simulink model "allmodes"  (Simulink 7.4)
settings: Solver=ode23tb  StartTime=0.0  StopTime=inf  MaxStep=1e-4  RelTol=1e-4
undefined symbols (not defined in the file): Ion, Lithium
libraries: powerlib x185, electricdrivelib x21, powerlib_extras x19, simulink x5
(part 5 of 7)

== system allmodes/vechicle units/vechicle-8 ==
  C1v8 : powerlib/Elements/Series RLC Branch  DialogController=POWERSYS.PowerSysDialog  PhysicalDomain=powersysdomain  SubClassName=unknown  LeftPortType=p1  RightPortType=p1  LConnTagsString=__new0  RConnTagsString=__new0  BranchType=C  Resistance=0.75  Inductance=1e-3  SetiL0=off  InitialCurrent=0  Capacitance=33e-6  Setx0=on  InitialVoltage=0  Measurements=Branch voltage and current
  Demux3 : Demux  Outputs=3
  Demux4 : Demux  Outputs=3
  IGBT20 : Subsystem
  IGBT21 : Subsystem
  L11v8 : powerlib/Elements/Series RLC Branch  DialogController=POWERSYS.PowerSysDialog  PhysicalDomain=powersysdomain  SubClassName=unknown  LeftPortType=p1  RightPortType=p1  LConnTagsString=__new0  RConnTagsString=__new0  BranchType=RL  Resistance=0.001  Inductance=0.0033  SetiL0=off  InitialCurrent=0  Capacitance=1e-6  Setx0=off  InitialVoltage=0  Measurements=Branch voltage and current
  L22v8 : powerlib/Elements/Series RLC Branch  DialogController=POWERSYS.PowerSysDialog  PhysicalDomain=powersysdomain  SubClassName=unknown  LeftPortType=p1  RightPortType=p1  LConnTagsString=__new0  RConnTagsString=__new0  BranchType=RL  Resistance=0.001  Inductance=1.2e-4  SetiL0=off  InitialCurrent=0  Capacitance=1e-6  Setx0=off  InitialVoltage=0  Measurements=Branch current
  Multimeter3 : powerlib/Measurements/Multimeter  SystemSampleTime=-1  PhasorSimulation=off  OutputType=Complex  sel=[41 112 113]  L=119  Gain=[1 1 1]  yselected={'Ub: vechicle units/vechicle-8/C1v8','Ib: vechicle units/vechicle-8/L11v8','Ib: vechicle units/vechicle-8/L22v8'};  PSBOutputType=1  PSBequivalent=0  AxesSetting=[0,0.1,-100,100]  Display=0  SavedBlockNames=-11
  v-8 : electricdrivelib/Extra Sources/Battery  DialogController=POWERSYS.PowerSysDialog  SystemSampleTime=-1  BatType=Lithium-Ion  ShowDetailedParameters=off  NomV=200  NomQ=30  SOC=50  PresetModel=on  MaxQ=30  FullV=232.7974  Dis_rate=13.0435  R=0.066667  Normal_OP=27.1304  expZone="[216.0772      1.473913]"  Dis_Char=off  current=[1.5 70]  Units=Ampere-hour  Batt_Tr=30
  +ve : PMIOPort  Port=1  Side=Left
  -ve : PMIOPort  Port=2  Side=Left
  tag scope: ISUIMv8=global, IbSUIMv8=global, Ibatv8=global, VbSUIMv8=global, VcSUIMv8=global, socv8=global
  wires:
  Demux3/1 -> [VcSUIMv8]
  Demux3/3 -> [IbSUIMv8]
  Demux3/2 -> [ISUIMv8]
  Multimeter3/1 -> Demux3/1
  Demux4/3 -> [VbSUIMv8]
  Demux4/2 -> [Ibatv8]
  Demux4/1 -> [socv8]
  v-8/1 -> Demux4/1
  connections:
  +ve/RConn1 -- IGBT20/RConn1
  L22v8/RConn1 -- v-8/LConn1
  IGBT21/RConn1 -- IGBT20/RConn2 -- L11v8/LConn1
  IGBT21/RConn2 -- -ve/RConn1 -- C1v8/RConn1 -- v-8/LConn2
  L11v8/RConn1 -- L22v8/LConn1 -- C1v8/LConn1

== system allmodes/vechicle units/vechicle-9 ==
  C1v9 : powerlib/Elements/Series RLC Branch  DialogController=POWERSYS.PowerSysDialog  PhysicalDomain=powersysdomain  SubClassName=unknown  LeftPortType=p1  RightPortType=p1  LConnTagsString=__new0  RConnTagsString=__new0  BranchType=C  Resistance=0.75  Inductance=1e-3  SetiL0=off  InitialCurrent=0  Capacitance=33e-6  Setx0=on  InitialVoltage=0  Measurements=Branch voltage and current
  Demux3 : Demux  Outputs=3
  Demux4 : Demux  Outputs=3
  IGBT20 : Subsystem
  IGBT21 : Subsystem
  L11v9 : powerlib/Elements/Series RLC Branch  DialogController=POWERSYS.PowerSysDialog  PhysicalDomain=powersysdomain  SubClassName=unknown  LeftPortType=p1  RightPortType=p1  LConnTagsString=__new0  RConnTagsString=__new0  BranchType=RL  Resistance=0.001  Inductance=0.0033  SetiL0=off  InitialCurrent=0  Capacitance=1e-6  Setx0=off  InitialVoltage=0  Measurements=Branch voltage and current
  L22v9 : powerlib/Elements/Series RLC Branch  DialogController=POWERSYS.PowerSysDialog  PhysicalDomain=powersysdomain  SubClassName=unknown  LeftPortType=p1  RightPortType=p1  LConnTagsString=__new0  RConnTagsString=__new0  BranchType=RL  Resistance=0.001  Inductance=1.2e-4  SetiL0=off  InitialCurrent=0  Capacitance=1e-6  Setx0=off  InitialVoltage=0  Measurements=Branch current
  Multimeter3 : powerlib/Measurements/Multimeter  SystemSampleTime=-1  PhasorSimulation=off  OutputType=Complex  sel=[43 115 116]  L=119  Gain=[1 1 1]  yselected={'Ub: vechicle units/vechicle-9/C1v9','Ib: vechicle units/vechicle-9/L11v9','Ib: vechicle units/vechicle-9/L22v9'};  PSBOutputType=1  PSBequivalent=0  AxesSetting=[0,0.1,-100,100]  Display=0  SavedBlockNames=-11
  v-9 : electricdrivelib/Extra Sources/Battery  DialogController=POWERSYS.PowerSysDialog  SystemSampleTime=-1  BatType=Lithium-Ion  ShowDetailedParameters=off  NomV=200  NomQ=30  SOC=50  PresetModel=on  MaxQ=30  FullV=232.7974  Dis_rate=13.0435  R=0.066667  Normal_OP=27.1304  expZone="[216.0772      1.473913]"  Dis_Char=off  current=[1.5 70]  Units=Ampere-hour  Batt_Tr=30
  +ve : PMIOPort  Port=1  Side=Left
  -ve : PMIOPort  Port=2  Side=Left
  tag scope: ISUIMv9=global, IbSUIMv9=global, Ibatv9=global, VbSUIMv9=global, VcSUIMv9=global, socv9=global
  wires:
  v-9/1 -> Demux4/1
  Demux4/1 -> [socv9]
  Demux4/2 -> [Ibatv9]
  Demux4/3 -> [VbSUIMv9]
  Multimeter3/1 -> Demux3/1
  Demux3/2 -> [ISUIMv9]
  Demux3/3 -> [IbSUIMv9]
  Demux3/1 -> [VcSUIMv9]
  connections:
  C1v9/LConn1 -- L22v9/LConn1 -- L11v9/RConn1
  v-9/LConn2 -- C1v9/RConn1 -- -ve/RConn1 -- IGBT21/RConn2
  L11v9/LConn1 -- IGBT20/RConn2 -- IGBT21/RConn1
  L22v9/RConn1 -- v-9/LConn1
  +ve/RConn1 -- IGBT20/RConn1

== system allmodes/CONTROLLER/AC/DC/AC controller/I-D REF ==
  Vdc_ref : Inport
  Vdc : Inport  Port=2
  Io : Inport  Port=3
  Gain1 : Gain  Gain=1/10  ParameterDataType=fixdt(1, 16)  ParameterScaling=2^0  OutDataType=fixdt(1, 16)  OutScaling=2^0
  Gain2 : Gain  Gain=1/0.7*0.25*0.5  ParameterDataType=fixdt(1, 16)  ParameterScaling=2^0  OutDataType=fixdt(1, 16)  OutScaling=2^0
  Gain3 : Gain  ParameterDataType=fixdt(1, 16)  ParameterScaling=2^0  OutDataType=fixdt(1, 16)  OutScaling=2^0
  Gain8 : Gain  Gain=10*5  ParameterDataType=fixdt(1, 16)  ParameterScaling=2^0  OutDataType=fixdt(1, 16)  OutScaling=2^0
  Integrator : Integrator
  Saturation : Saturate  UpperLimit=10000  LowerLimit=-10000  OutDataType=fixdt(1, 16)  OutScaling=2^0
  Sum : Sum  Inputs=+|+|+  OutDataType=fixdt(1, 16)  OutScaling=2^0
  Sum1 : Sum  Inputs=|+-  OutDataType=fixdt(1, 16)  OutScaling=2^0
  Sum3 : Sum  Inputs=|+-  OutDataType=fixdt(1, 16)  OutScaling=2^0
  Sum4 : Sum  Inputs=++|  OutDataType=fixdt(1, 16)  OutScaling=2^0
  Id_ref : Outport
  wires:
  Sum1/1 -> Gain8/1, Sum4/2
  Sum/1 -> Sum3/2, Saturation/1
  Vdc_ref/1 -> Sum1/1
  Vdc/1 -> Sum1/2
  Saturation/1 -> Id_ref/1, Sum3/1
  Sum3/1 -> Gain1/1
  Gain1/1 -> Sum4/1
  Integrator/1 -> Sum/2
  Gain8/1 -> Sum/3
  Gain2/1 -> Sum/1
  Gain3/1 -> Integrator/1
  Sum4/1 -> Gain3/1
  Io/1 -> Gain2/1

== system allmodes/CONTROLLER/AC/DC/AC controller/abc-dq ==
  In1 : Inport
  Demux : Demux  Outputs=3
  Discrete Virtual PLL : powerlib_extras/Discrete  Control Blocks/Discrete Virtual PLL  DialogController=POWERSYS.PowerSysDialog  SystemSampleTime=-1  Freq=60  Phase=0  Ts=50e-6
  Mux : Mux  Inputs=2
  abc_to_dq0 ransformation : powerlib_extras/Measurements/abc_to_dq0 Transformation  DialogController=POWERSYS.PowerSysDialog  SystemSampleTime=-1
  d : Outport
  wires:
  In1/1 -> abc_to_dq0 ransformation/1
  Discrete Virtual PLL/2 -> abc_to_dq0 ransformation/2
  abc_to_dq0 ransformation/1 -> Demux/1
  Demux/1 -> Mux/1
  Demux/2 -> Mux/2
  Mux/1 -> d/1

== system allmodes/CONTROLLER/AC/DC/AC controller/abc-dq2 ==
  In1 : Inport
  Demux : Demux  Outputs=3
  Discrete Virtual PLL : powerlib_extras/Discrete  Control Blocks/Discrete Virtual PLL  DialogController=POWERSYS.PowerSysDialog  SystemSampleTime=-1  Freq=60  Phase=0  Ts=50e-6
  Mux : Mux  Inputs=2
  abc_to_dq0 ransformation : powerlib_extras/Measurements/abc_to_dq0 Transformation  DialogController=POWERSYS.PowerSysDialog  SystemSampleTime=-1
  d : Outport
  wires:
  In1/1 -> abc_to_dq0 ransformation/1
  Discrete Virtual PLL/2 -> abc_to_dq0 ransformation/2
  abc_to_dq0 ransformation/1 -> Demux/1
  Demux/1 -> Mux/1
  Demux/2 -> Mux/2
  Mux/1 -> d/1

== system allmodes/CONTROLLER/AC/DC/AC controller/abc-dq4 ==
  In1 : Inport
  Demux1 : Demux  Outputs=2
  Discrete Virtual PLL : powerlib_extras/Discrete  Control Blocks/Discrete Virtual PLL  DialogController=POWERSYS.PowerSysDialog  SystemSampleTime=-1  Freq=60  Phase=0  Ts=50e-6
  Mux1 : Mux  Inputs=3
  dq0_to_abc Transformation : powerlib_extras/Measurements/dq0_to_abc Transformation  DialogController=POWERSYS.PowerSysDialog  SystemSampleTime=-1
  q : Outport
  wires:
  Discrete Virtual PLL/2 -> dq0_to_abc Transformation/2
  Mux1/1 -> dq0_to_abc Transformation/1
  Demux1/1 -> Mux1/1
  Demux1/2 -> Mux1/2
  In1/1 -> Demux1/1
  dq0_to_abc Transformation/1 -> q/1

== system allmodes/CONTROLLER/AC/DC/AC controller/current  controller ==
  Id_ref : Inport
  Idq : Inport  Port=2
  Vc_dq : Inport  Port=3
  Vdc : Inport  Port=4
  Complex to Magnitude-Angle : ComplexToMagnitudeAngle
  Complex to Real-Imag : ComplexToRealImag
  Constant2 : Constant  Value=0  OutDataType=fixdt(1, 16)  OutScaling=2^0
  Demux1 : Demux  Outputs=2
  Divide1 : Product  Inputs=*/  OutDataType=fixdt(1, 16)  OutScaling=2^-10
  Divide2 : Product  Inputs=**  OutDataType=fixdt(1, 16)  OutScaling=2^-10
  Gain1 : Gain  Gain=314.1593*5e-4*[-1 1]  ParameterDataType=fixdt(1, 16)  ParameterScaling=2^0  OutDataType=fixdt(1, 16)  OutScaling=2^0
  Gain2 : Gain  Gain=0.03  ParameterDataType=fixdt(1, 16)  ParameterScaling=2^0  OutDataType=fixdt(1, 16)  OutScaling=2^0
  Gain3 : Gain  Gain=[1 1j]  Multiplication=Matrix(K*u) (u vector)  ParameterDataType=fixdt(1, 16)  ParameterScaling=2^0  OutDataType=fixdt(1, 16)  OutScaling=2^0
  Gain4 : Gain  Gain=1/2  ParameterDataType=fixdt(1, 16)  ParameterScaling=2^0  OutDataType=fixdt(1, 16)  OutScaling=2^0
  Gain5 : Gain  Gain=155  ParameterDataType=fixdt(1, 16)  ParameterScaling=2^0  OutDataType=fixdt(1, 16)  OutScaling=2^0
  Gain7 : Gain  Gain=1/2.5  ParameterDataType=fixdt(1, 16)  ParameterScaling=2^0  OutDataType=fixdt(1, 16)  OutScaling=2^0
  Gain8 : Gain  Gain=2.5  ParameterDataType=fixdt(1, 16)  ParameterScaling=2^0  OutDataType=fixdt(1, 16)  OutScaling=2^0
  Integrator : Integrator
  Magnitude-Angle to Complex : MagnitudeAngleToComplex
  Mux : Mux  Inputs=2
  Mux1 : Mux  Inputs=2
  Mux2 : Mux  Inputs=2
  Saturation : Saturate  UpperLimit=4  LowerLimit=-4  OutDataType=fixdt(1, 16)  OutScaling=2^0
  Sum : Sum  Inputs=|++  OutDataType=fixdt(1, 16)  OutScaling=2^0
  Sum1 : Sum  Inputs=|++  OutDataType=fixdt(1, 16)  OutScaling=2^0
  Sum2 : Sum  Inputs=|-|++  OutDataType=fixdt(1, 16)  OutScaling=2^0
  Sum3 : Sum  Inputs=|+-  OutDataType=fixdt(1, 16)  OutScaling=2^0
  Sum6 : Sum  Inputs=|-+  OutDataType=fixdt(1, 16)  OutScaling=2^0
  Sum8 : Sum  Inputs=++|  OutDataType=fixdt(1, 16)  OutScaling=2^0
  Vi_dq_ref : Outport
  wires:
  Idq/1 -> Gain1/1, Gain2/1, Sum3/2
  Vc_dq/1 -> Sum1/2
  Sum3/1 -> Gain8/1, Sum8/2
  Sum/1 -> Sum2/1
  Mux/1 -> Sum3/1
  Gain1/1 -> Demux1/1
  Demux1/2 -> Mux1/1
  Demux1/1 -> Mux1/2
  Complex to Magnitude-Angle/1 -> Saturation/1
  Saturation/1 -> Magnitude-Angle to Complex/1
  Complex to Magnitude-Angle/2 -> Magnitude-Angle to Complex/2
  Magnitude-Angle to Complex/1 -> Complex to Real-Imag/1
  Complex to Real-Imag/1 -> Mux2/1
  Complex to Real-Imag/2 -> Mux2/2
  Mux2/1 -> Sum6/1, Vi_dq_ref/1
  Gain8/1 -> Sum/2
  Mux1/1 -> Sum1/1
  Id_ref/1 -> Mux/1
  Gain3/1 -> Complex to Magnitude-Angle/1
  Vdc/1 -> Gain4/1
  Sum2/1 -> Divide1/1
  Divide1/1 -> Sum6/2, Gain3/1
  Gain7/1 -> Sum8/1
  Divide2/1 -> Gain7/1
  Sum6/1 -> Divide2/1
  Gain4/1 -> Divide1/2, Divide2/2
  Gain2/1 -> Sum2/2
  Sum1/1 -> Sum2/3
  Constant2/1 -> Mux/2
  Gain5/1 -> Integrator/1
  Integrator/1 -> Sum/1
  Sum8/1 -> Gain5/1

== system allmodes/CONTROLLER/AC/DC/AC controller1/I-D REF ==
  Vdc_ref : Inport
  Vdc : Inport  Port=2
  Io : Inport  Port=3
  Gain1 : Gain  Gain=1/10  ParameterDataType=fixdt(1, 16)  ParameterScaling=2^0  OutDataType=fixdt(1, 16)  OutScaling=2^0
  Gain2 : Gain  Gain=1/0.7*0.25*0.5  ParameterDataType=fixdt(1, 16)  ParameterScaling=2^0  OutDataType=fixdt(1, 16)  OutScaling=2^0
  Gain3 : Gain  ParameterDataType=fixdt(1, 16)  ParameterScaling=2^0  OutDataType=fixdt(1, 16)  OutScaling=2^0
  Gain8 : Gain  Gain=10*5  ParameterDataType=fixdt(1, 16)  ParameterScaling=2^0  OutDataType=fixdt(1, 16)  OutScaling=2^0
  Integrator : Integrator
  Saturation : Saturate  UpperLimit=10000  LowerLimit=-10000  OutDataType=fixdt(1, 16)  OutScaling=2^0
  Sum : Sum  Inputs=+|+|+  OutDataType=fixdt(1, 16)  OutScaling=2^0
  Sum1 : Sum  Inputs=|+-  OutDataType=fixdt(1, 16)  OutScaling=2^0
  Sum3 : Sum  Inputs=|+-  OutDataType=fixdt(1, 16)  OutScaling=2^0
  Sum4 : Sum  Inputs=++|  OutDataType=fixdt(1, 16)  OutScaling=2^0
  Id_ref : Outport
  wires:
  Sum4/1 -> Gain3/1
  Gain3/1 -> Integrator/1
  Gain2/1 -> Sum/1
  Gain8/1 -> Sum/3
  Integrator/1 -> Sum/2
  Io/1 -> Gain2/1
  Gain1/1 -> Sum4/1
  Sum3/1 -> Gain1/1
  Saturation/1 -> Sum3/1, Id_ref/1
  Vdc/1 -> Sum1/2
  Vdc_ref/1 -> Sum1/1
  Sum/1 -> Saturation/1, Sum3/2
  Sum1/1 -> Sum4/2, Gain8/1

== system allmodes/CONTROLLER/AC/DC/AC controller1/abc-dq ==
  In1 : Inport
  Demux : Demux  Outputs=3
  Discrete Virtual PLL : powerlib_extras/Discrete  Control Blocks/Discrete Virtual PLL  DialogController=POWERSYS.PowerSysDialog  SystemSampleTime=-1  Freq=60  Phase=0  Ts=50e-6
  Mux : Mux  Inputs=2
  abc_to_dq0 ransformation : powerlib_extras/Measurements/abc_to_dq0 Transformation  DialogController=POWERSYS.PowerSysDialog  SystemSampleTime=-1
  d : Outport
  wires:
  Mux/1 -> d/1
  Demux/2 -> Mux/2
  Demux/1 -> Mux/1
  abc_to_dq0 ransformation/1 -> Demux/1
  Discrete Virtual PLL/2 -> abc_to_dq0 ransformation/2
  In1/1 -> abc_to_dq0 ransformation/1

== system allmodes/CONTROLLER/AC/DC/AC controller1/abc-dq2 ==
  In1 : Inport
  Demux : Demux  Outputs=3
  Discrete Virtual PLL : powerlib_extras/Discrete  Control Blocks/Discrete Virtual PLL  DialogController=POWERSYS.PowerSysDialog  SystemSampleTime=-1  Freq=60  Phase=0  Ts=50e-6
  Mux : Mux  Inputs=2
  abc_to_dq0 ransformation : powerlib_extras/Measurements/abc_to_dq0 Transformation  DialogController=POWERSYS.PowerSysDialog  SystemSampleTime=-1
  d : Outport
  wires:
  Mux/1 -> d/1
  Demux/2 -> Mux/2
  Demux/1 -> Mux/1
  abc_to_dq0 ransformation/1 -> Demux/1
  Discrete Virtual PLL/2 -> abc_to_dq0 ransformation/2
  In1/1 -> abc_to_dq0 ransformation/1

== system allmodes/CONTROLLER/AC/DC/AC controller1/abc-dq4 ==
  In1 : Inport
  Demux1 : Demux  Outputs=2
  Discrete Virtual PLL : powerlib_extras/Discrete  Control Blocks/Discrete Virtual PLL  DialogController=POWERSYS.PowerSysDialog  SystemSampleTime=-1  Freq=60  Phase=0  Ts=50e-6
  Mux1 : Mux  Inputs=3
  dq0_to_abc Transformation : powerlib_extras/Measurements/dq0_to_abc Transformation  DialogController=POWERSYS.PowerSysDialog  SystemSampleTime=-1
  q : Outport
  wires:
  dq0_to_abc Transformation/1 -> q/1
  In1/1 -> Demux1/1
  Demux1/2 -> Mux1/2
  Demux1/1 -> Mux1/1
  Mux1/1 -> dq0_to_abc Transformation/1
  Discrete Virtual PLL/2 -> dq0_to_abc Transformation/2

== system allmodes/CONTROLLER/AC/DC/AC controller1/current  controller ==
  Id_ref : Inport
  Idq : Inport  Port=2
  Vc_dq : Inport  Port=3
  Vdc : Inport  Port=4
  Complex to Magnitude-Angle : ComplexToMagnitudeAngle
  Complex to Real-Imag : ComplexToRealImag
  Constant2 : Constant  Value=0  OutDataType=fixdt(1, 16)  OutScaling=2^0
  Demux1 : Demux  Outputs=2
  Divide1 : Product  Inputs=*/  OutDataType=fixdt(1, 16)  OutScaling=2^-10
  Divide2 : Product  Inputs=**  OutDataType=fixdt(1, 16)  OutScaling=2^-10
  Gain1 : Gain  Gain=314.1593*5e-4*[-1 1]  ParameterDataType=fixdt(1, 16)  ParameterScaling=2^0  OutDataType=fixdt(1, 16)  OutScaling=2^0
  Gain2 : Gain  Gain=0.03  ParameterDataType=fixdt(1, 16)  ParameterScaling=2^0  OutDataType=fixdt(1, 16)  OutScaling=2^0
  Gain3 : Gain  Gain=[1 1j]  Multiplication=Matrix(K*u) (u vector)  ParameterDataType=fixdt(1, 16)  ParameterScaling=2^0  OutDataType=fixdt(1, 16)  OutScaling=2^0
  Gain4 : Gain  Gain=1/2  ParameterDataType=fixdt(1, 16)  ParameterScaling=2^0  OutDataType=fixdt(1, 16)  OutScaling=2^0
  Gain5 : Gain  Gain=155  ParameterDataType=fixdt(1, 16)  ParameterScaling=2^0  OutDataType=fixdt(1, 16)  OutScaling=2^0
  Gain7 : Gain  Gain=1/2.5  ParameterDataType=fixdt(1, 16)  ParameterScaling=2^0  OutDataType=fixdt(1, 16)  OutScaling=2^0
  Gain8 : Gain  Gain=2.5  ParameterDataType=fixdt(1, 16)  ParameterScaling=2^0  OutDataType=fixdt(1, 16)  OutScaling=2^0
  Integrator : Integrator
  Magnitude-Angle to Complex : MagnitudeAngleToComplex
  Mux : Mux  Inputs=2
  Mux1 : Mux  Inputs=2
  Mux2 : Mux  Inputs=2
  Saturation : Saturate  UpperLimit=4  LowerLimit=-4  OutDataType=fixdt(1, 16)  OutScaling=2^0
  Sum : Sum  Inputs=|++  OutDataType=fixdt(1, 16)  OutScaling=2^0
  Sum1 : Sum  Inputs=|++  OutDataType=fixdt(1, 16)  OutScaling=2^0
  Sum2 : Sum  Inputs=|-|++  OutDataType=fixdt(1, 16)  OutScaling=2^0
  Sum3 : Sum  Inputs=|+-  OutDataType=fixdt(1, 16)  OutScaling=2^0
  Sum6 : Sum  Inputs=|-+  OutDataType=fixdt(1, 16)  OutScaling=2^0
  Sum8 : Sum  Inputs=++|  OutDataType=fixdt(1, 16)  OutScaling=2^0
  Vi_dq_ref : Outport
  wires:
  Idq/1 -> Gain1/1, Gain2/1, Sum3/2
  Vc_dq/1 -> Sum1/2
  Sum3/1 -> Gain8/1, Sum8/2
  Sum/1 -> Sum2/1
  Mux/1 -> Sum3/1
  Gain1/1 -> Demux1/1
  Demux1/2 -> Mux1/1
  Demux1/1 -> Mux1/2
  Complex to Magnitude-Angle/1 -> Saturation/1
  Saturation/1 -> Magnitude-Angle to Complex/1
  Complex to Magnitude-Angle/2 -> Magnitude-Angle to Complex/2
  Magnitude-Angle to Complex/1 -> Complex to Real-Imag/1
  Complex to Real-Imag/1 -> Mux2/1
  Complex to Real-Imag/2 -> Mux2/2
  Mux2/1 -> Sum6/1, Vi_dq_ref/1
  Gain8/1 -> Sum/2
  Mux1/1 -> Sum1/1
  Id_ref/1 -> Mux/1
  Gain3/1 -> Complex to Magnitude-Angle/1
  Vdc/1 -> Gain4/1
  Sum2/1 -> Divide1/1
  Divide1/1 -> Sum6/2, Gain3/1
  Gain7/1 -> Sum8/1
  Divide2/1 -> Gain7/1
  Sum6/1 -> Divide2/1
  Gain4/1 -> Divide1/2, Divide2/2
  Gain2/1 -> Sum2/2
  Sum1/1 -> Sum2/3
  Constant2/1 -> Mux/2
  Gain5/1 -> Integrator/1
  Integrator/1 -> Sum/1
  Sum8/1 -> Gain5/1

== system allmodes/CONTROLLER/AC/DC/AC controller2/I-D REF ==
  Vdc_ref : Inport
  Vdc : Inport  Port=2
  Io : Inport  Port=3
  Gain1 : Gain  Gain=1/10  ParameterDataType=fixdt(1, 16)  ParameterScaling=2^0  OutDataType=fixdt(1, 16)  OutScaling=2^0
  Gain2 : Gain  Gain=1/0.7*0.25*0.5  ParameterDataType=fixdt(1, 16)  ParameterScaling=2^0  OutDataType=fixdt(1, 16)  OutScaling=2^0
  Gain3 : Gain  ParameterDataType=fixdt(1, 16)  ParameterScaling=2^0  OutDataType=fixdt(1, 16)  OutScaling=2^0
  Gain8 : Gain  Gain=10*5  ParameterDataType=fixdt(1, 16)  ParameterScaling=2^0  OutDataType=fixdt(1, 16)  OutScaling=2^0
  Integrator : Integrator
  Saturation : Saturate  UpperLimit=10000  LowerLimit=-10000  OutDataType=fixdt(1, 16)  OutScaling=2^0
  Sum : Sum  Inputs=+|+|+  OutDataType=fixdt(1, 16)  OutScaling=2^0
  Sum1 : Sum  Inputs=|+-  OutDataType=fixdt(1, 16)  OutScaling=2^0
  Sum3 : Sum  Inputs=|+-  OutDataType=fixdt(1, 16)  OutScaling=2^0
  Sum4 : Sum  Inputs=++|  OutDataType=fixdt(1, 16)  OutScaling=2^0
  Id_ref : Outport
  wires:
  Sum1/1 -> Gain8/1, Sum4/2
  Sum/1 -> Sum3/2, Saturation/1
  Vdc_ref/1 -> Sum1/1
  Vdc/1 -> Sum1/2
  Saturation/1 -> Id_ref/1, Sum3/1
  Sum3/1 -> Gain1/1
  Gain1/1 -> Sum4/1
  Io/1 -> Gain2/1
  Integrator/1 -> Sum/2
  Gain8/1 -> Sum/3
  Gain2/1 -> Sum/1
  Gain3/1 -> Integrator/1
  Sum4/1 -> Gain3/1

== system allmodes/CONTROLLER/AC/DC/AC controller2/abc-dq ==
  In1 : Inport
  Demux : Demux  Outputs=3
  Discrete Virtual PLL : powerlib_extras/Discrete  Control Blocks/Discrete Virtual PLL  DialogController=POWERSYS.PowerSysDialog  SystemSampleTime=-1  Freq=60  Phase=0  Ts=50e-6
  Mux : Mux  Inputs=2
  abc_to_dq0 ransformation : powerlib_extras/Measurements/abc_to_dq0 Transformation  DialogController=POWERSYS.PowerSysDialog  SystemSampleTime=-1
  d : Outport
  wires:
  In1/1 -> abc_to_dq0 ransformation/1
  Discrete Virtual PLL/2 -> abc_to_dq0 ransformation/2
  abc_to_dq0 ransformation/1 -> Demux/1
  Demux/1 -> Mux/1
  Demux/2 -> Mux/2
  Mux/1 -> d/1

== system allmodes/CONTROLLER/AC/DC/AC controller2/abc-dq2 ==
  In1 : Inport
  Demux : Demux  Outputs=3
  Discrete Virtual PLL : powerlib_extras/Discrete  Control Blocks/Discrete Virtual PLL  DialogController=POWERSYS.PowerSysDialog  SystemSampleTime=-1  Freq=60  Phase=0  Ts=50e-6
  Mux : Mux  Inputs=2
  abc_to_dq0 ransformation : powerlib_extras/Measurements/abc_to_dq0 Transformation  DialogController=POWERSYS.PowerSysDialog  SystemSampleTime=-1
  d : Outport
  wires:
  In1/1 -> abc_to_dq0 ransformation/1
  Discrete Virtual PLL/2 -> abc_to_dq0 ransformation/2
  abc_to_dq0 ransformation/1 -> Demux/1
  Demux/1 -> Mux/1
  Demux/2 -> Mux/2
  Mux/1 -> d/1

== system allmodes/CONTROLLER/AC/DC/AC controller2/abc-dq4 ==
  In1 : Inport
  Demux1 : Demux  Outputs=2
  Discrete Virtual PLL : powerlib_extras/Discrete  Control Blocks/Discrete Virtual PLL  DialogController=POWERSYS.PowerSysDialog  SystemSampleTime=-1  Freq=60  Phase=0  Ts=50e-6
  Mux1 : Mux  Inputs=3
  dq0_to_abc Transformation : powerlib_extras/Measurements/dq0_to_abc Transformation  DialogController=POWERSYS.PowerSysDialog  SystemSampleTime=-1
  q : Outport
  wires:
  Discrete Virtual PLL/2 -> dq0_to_abc Transformation/2
  Mux1/1 -> dq0_to_abc Transformation/1
  Demux1/1 -> Mux1/1
  Demux1/2 -> Mux1/2
  In1/1 -> Demux1/1
  dq0_to_abc Transformation/1 -> q/1

== system allmodes/CONTROLLER/AC/DC/AC controller2/current  controller ==
  Id_ref : Inport
  Idq : Inport  Port=2
  Vc_dq : Inport  Port=3
  Vdc : Inport  Port=4
  Complex to Magnitude-Angle : ComplexToMagnitudeAngle
  Complex to Real-Imag : ComplexToRealImag
  Constant2 : Constant  Value=0  OutDataType=fixdt(1, 16)  OutScaling=2^0
  Demux1 : Demux  Outputs=2
  Divide1 : Product  Inputs=*/  OutDataType=fixdt(1, 16)  OutScaling=2^-10
  Divide2 : Product  Inputs=**  OutDataType=fixdt(1, 16)  OutScaling=2^-10
  Gain1 : Gain  Gain=314.1593*5e-4*[-1 1]  ParameterDataType=fixdt(1, 16)  ParameterScaling=2^0  OutDataType=fixdt(1, 16)  OutScaling=2^0
  Gain2 : Gain  Gain=0.03  ParameterDataType=fixdt(1, 16)  ParameterScaling=2^0  OutDataType=fixdt(1, 16)  OutScaling=2^0
  Gain3 : Gain  Gain=[1 1j]  Multiplication=Matrix(K*u) (u vector)  ParameterDataType=fixdt(1, 16)  ParameterScaling=2^0  OutDataType=fixdt(1, 16)  OutScaling=2^0
  Gain4 : Gain  Gain=1/2  ParameterDataType=fixdt(1, 16)  ParameterScaling=2^0  OutDataType=fixdt(1, 16)  OutScaling=2^0
  Gain5 : Gain  Gain=155  ParameterDataType=fixdt(1, 16)  ParameterScaling=2^0  OutDataType=fixdt(1, 16)  OutScaling=2^0
  Gain7 : Gain  Gain=1/2.5  ParameterDataType=fixdt(1, 16)  ParameterScaling=2^0  OutDataType=fixdt(1, 16)  OutScaling=2^0
  Gain8 : Gain  Gain=2.5  ParameterDataType=fixdt(1, 16)  ParameterScaling=2^0  OutDataType=fixdt(1, 16)  OutScaling=2^0
  Integrator : Integrator
  Magnitude-Angle to Complex : MagnitudeAngleToComplex
  Mux : Mux  Inputs=2
  Mux1 : Mux  Inputs=2
  Mux2 : Mux  Inputs=2
  Saturation : Saturate  UpperLimit=4  LowerLimit=-4  OutDataType=fixdt(1, 16)  OutScaling=2^0
  Sum : Sum  Inputs=|++  OutDataType=fixdt(1, 16)  OutScaling=2^0
  Sum1 : Sum  Inputs=|++  OutDataType=fixdt(1, 16)  OutScaling=2^0
  Sum2 : Sum  Inputs=|-|++  OutDataType=fixdt(1, 16)  OutScaling=2^0
  Sum3 : Sum  Inputs=|+-  OutDataType=fixdt(1, 16)  OutScaling=2^0
  Sum6 : Sum  Inputs=|-+  OutDataType=fixdt(1, 16)  OutScaling=2^0
  Sum8 : Sum  Inputs=++|  OutDataType=fixdt(1, 16)  OutScaling=2^0
  Vi_dq_ref : Outport
  wires:
  Idq/1 -> Gain1/1, Gain2/1, Sum3/2
  Vc_dq/1 -> Sum1/2
  Sum3/1 -> Gain8/1, Sum8/2
  Sum/1 -> Sum2/1
  Mux/1 -> Sum3/1
  Gain1/1 -> Demux1/1
  Demux1/2 -> Mux1/1
  Demux1/1 -> Mux1/2
  Complex to Magnitude-Angle/1 -> Saturation/1
  Saturation/1 -> Magnitude-Angle to Complex/1
  Complex to Magnitude-Angle/2 -> Magnitude-Angle to Complex/2
  Magnitude-Angle to Complex/1 -> Complex to Real-Imag/1
  Complex to Real-Imag/1 -> Mux2/1
  Complex to Real-Imag/2 -> Mux2/2
  Mux2/1 -> Sum6/1, Vi_dq_ref/1
  Gain8/1 -> Sum/2
  Mux1/1 -> Sum1/1
  Id_ref/1 -> Mux/1
  Gain3/1 -> Complex to Magnitude-Angle/1
  Vdc/1 -> Gain4/1
  Sum2/1 -> Divide1/1
  Divide1/1 -> Sum6/2, Gain3/1
  Gain7/1 -> Sum8/1
  Divide2/1 -> Gain7/1
  Sum6/1 -> Divide2/1
  Gain4/1 -> Divide1/2, Divide2/2
  Gain2/1 -> Sum2/2
  Sum1/1 -> Sum2/3
  Constant2/1 -> Mux/2
  Gain5/1 -> Integrator/1
  Integrator/1 -> Sum/1
  Sum8/1 -> Gain5/1

== system allmodes/CONTROLLER/RECTIFIER1/triangular wave gen1 ==
  Clock : Clock
      settings: Decimation=10
  Constant : Constant  Value=1/fsw  OutDataType=fixdt(1, 16)  OutScaling=2^0
  Constant1 : Constant  OutDataType=fixdt(1, 16)  OutScaling=2^0
  Constant2 : Constant  Value=3  OutDataType=fixdt(1, 16)  OutScaling=2^0
  Divide : Product  Inputs=*/  OutDataType=fixdt(1, 16)  OutScaling=2^-10
  Divide1 : Product  Inputs=/*  OutDataType=fixdt(1, 16)  OutScaling=2^-10
  Gain1 : Gain  Gain=0.25  ParameterDataType=fixdt(1, 16)  ParameterScaling=2^0  OutDataType=fixdt(1, 16)  OutScaling=2^0
  Gain2 : Gain  Gain=4  ParameterDataType=fixdt(1, 16)  ParameterScaling=2^0  OutDataType=fixdt(1, 16)  OutScaling=2^0
  Gain3 : Gain  Gain=mag  ParameterDataType=fixdt(1, 16)  ParameterScaling=2^0  OutDataType=fixdt(1, 16)  OutScaling=2^0
  Math Function : Math  Operator=rem  OutDataType=fixdt(1, 16)  OutScaling=2^0  SaturateOnIntegerOverflow=on
  Sum1 : Sum  Inputs=+|+  OutDataType=fixdt(1, 16)  OutScaling=2^0
  Sum3 : Sum  Inputs=|+-  OutDataType=fixdt(1, 16)  OutScaling=2^0
  Sum4 : Sum  Inputs=|-+  OutDataType=fixdt(1, 16)  OutScaling=2^0
  Switch : Switch  Threshold=1/(2*fsw)  OutDataType=fixdt(1, 16)  OutScaling=2^0
  tri_out : Outport
  wires:
  Constant/1 -> Math Function/2, Divide1/1, Divide/2, Gain1/1
  Math Function/1 -> Switch/2, Gain2/1
  Sum3/1 -> Switch/3
  Divide1/1 -> Sum4/1
  Constant2/1 -> Sum4/2
  Sum4/1 -> Switch/1
  Divide/1 -> Sum3/1
  Constant1/1 -> Sum3/2
  Switch/1 -> Gain3/1
  Clock/1 -> Sum1/1
  Sum1/1 -> Math Function/1
  Gain2/1 -> Divide1/2, Divide/1
  Gain1/1 -> Sum1/2
  Gain3/1 -> tri_out/1

== system allmodes/CONTROLLER/RECTIFIER2/triangular wave gen1 ==
  Clock : Clock
      settings: Decimation=10
  Constant : Constant  Value=1/fsw  OutDataType=fixdt(1, 16)  OutScaling=2^0
  Constant1 : Constant  OutDataType=fixdt(1, 16)  OutScaling=2^0
  Constant2 : Constant  Value=3  OutDataType=fixdt(1, 16)  OutScaling=2^0
  Divide : Product  Inputs=*/  OutDataType=fixdt(1, 16)  OutScaling=2^-10
  Divide1 : Product  Inputs=/*  OutDataType=fixdt(1, 16)  OutScaling=2^-10
  Gain1 : Gain  Gain=0.25  ParameterDataType=fixdt(1, 16)  ParameterScaling=2^0  OutDataType=fixdt(1, 16)  OutScaling=2^0
  Gain2 : Gain  Gain=4  ParameterDataType=fixdt(1, 16)  ParameterScaling=2^0  OutDataType=fixdt(1, 16)  OutScaling=2^0
  Gain3 : Gain  Gain=mag  ParameterDataType=fixdt(1, 16)  ParameterScaling=2^0  OutDataType=fixdt(1, 16)  OutScaling=2^0
  Math Function : Math  Operator=rem  OutDataType=fixdt(1, 16)  OutScaling=2^0  SaturateOnIntegerOverflow=on
  Sum1 : Sum  Inputs=+|+  OutDataType=fixdt(1, 16)  OutScaling=2^0
  Sum3 : Sum  Inputs=|+-  OutDataType=fixdt(1, 16)  OutScaling=2^0
  Sum4 : Sum  Inputs=|-+  OutDataType=fixdt(1, 16)  OutScaling=2^0
  Switch : Switch  Threshold=1/(2*fsw)  OutDataType=fixdt(1, 16)  OutScaling=2^0
  tri_out : Outport
  wires:
  Gain3/1 -> tri_out/1
  Gain1/1 -> Sum1/2
  Gain2/1 -> Divide/1, Divide1/2
  Sum1/1 -> Math Function/1
  Clock/1 -> Sum1/1
  Switch/1 -> Gain3/1
  Constant1/1 -> Sum3/2
  Divide/1 -> Sum3/1
  Sum4/1 -> Switch/1
  Constant2/1 -> Sum4/2
  Divide1/1 -> Sum4/1
  Sum3/1 -> Switch/3
  Math Function/1 -> Gain2/1, Switch/2
  Constant/1 -> Gain1/1, Divide/2, Divide1/1, Math Function/2

== system allmodes/CONTROLLER/RECTIFIER3/triangular wave gen1 ==
  Clock : Clock
      settings: Decimation=10
  Constant : Constant  Value=1/fsw  OutDataType=fixdt(1, 16)  OutScaling=2^0
  Constant1 : Constant  OutDataType=fixdt(1, 16)  OutScaling=2^0
  Constant2 : Constant  Value=3  OutDataType=fixdt(1, 16)  OutScaling=2^0
  Divide : Product  Inputs=*/  OutDataType=fixdt(1, 16)  OutScaling=2^-10
  Divide1 : Product  Inputs=/*  OutDataType=fixdt(1, 16)  OutScaling=2^-10
  Gain1 : Gain  Gain=0.25  ParameterDataType=fixdt(1, 16)  ParameterScaling=2^0  OutDataType=fixdt(1, 16)  OutScaling=2^0
  Gain2 : Gain  Gain=4  ParameterDataType=fixdt(1, 16)  ParameterScaling=2^0  OutDataType=fixdt(1, 16)  OutScaling=2^0
  Gain3 : Gain  Gain=mag  ParameterDataType=fixdt(1, 16)  ParameterScaling=2^0  OutDataType=fixdt(1, 16)  OutScaling=2^0
  Math Function : Math  Operator=rem  OutDataType=fixdt(1, 16)  OutScaling=2^0  SaturateOnIntegerOverflow=on
  Sum1 : Sum  Inputs=+|+  OutDataType=fixdt(1, 16)  OutScaling=2^0
  Sum3 : Sum  Inputs=|+-  OutDataType=fixdt(1, 16)  OutScaling=2^0
  Sum4 : Sum  Inputs=|-+  OutDataType=fixdt(1, 16)  OutScaling=2^0
  Switch : Switch  Threshold=1/(2*fsw)  OutDataType=fixdt(1, 16)  OutScaling=2^0
  tri_out : Outport
  wires:
  Constant/1 -> Math Function/2, Divide1/1, Divide/2, Gain1/1
  Math Function/1 -> Switch/2, Gain2/1
  Sum3/1 -> Switch/3
  Divide1/1 -> Sum4/1
  Constant2/1 -> Sum4/2
  Sum4/1 -> Switch/1
  Divide/1 -> Sum3/1
  Constant1/1 -> Sum3/2
  Switch/1 -> Gain3/1
  Clock/1 -> Sum1/1
  Sum1/1 -> Math Function/1
  Gain2/1 -> Divide1/2, Divide/1
  Gain1/1 -> Sum1/2
  Gain3/1 -> tri_out/1

== system allmodes/battery controller /SUIM1/Subsystem ==
  In1 : Inport
  Enable : EnablePort
  Constant2 : Constant  Value=0  OutDataType=fixdt(1, 16)  OutScaling=2^0
  Data Type Conversion2 : DataTypeConversion  OutDataType=fixdt(1, 16)  OutScaling=2^0
  Data Type Conversion3 : DataTypeConversion  OutDataType=fixdt(1, 16)  OutScaling=2^0
  Gain1 : Gain  Gain=-1  ParameterDataType=fixdt(1, 16)  ParameterScaling=2^0  OutDataType=fixdt(1, 16)  OutScaling=2^0
  Relational Operator2 : RelationalOperator  Operator=>  LogicOutDataTypeMode=boolean  LogicDataType=fixdt(0, 8)  OutDataTypeStr=boolean
  Relational Operator3 : RelationalOperator  Operator=>  LogicOutDataTypeMode=boolean  LogicDataType=fixdt(0, 8)  OutDataTypeStr=boolean
  Switch1 : Switch  OutDataType=fixdt(1, 16)  OutScaling=2^0
  Switch2 : Switch  Criteria=u2 > Threshold  OutDataType=fixdt(1, 16)  OutScaling=2^0
  sawtooth generator : Subsystem  mask{fsw=5e3, vc=1}
      mask prompts: fsw "switching frequency"; vc "magnitude"
  Out1 : Outport
  Out2 : Outport  Port=2
  wires:
  Relational Operator3/1 -> Data Type Conversion2/1
  Relational Operator2/1 -> Data Type Conversion3/1
  Data Type Conversion3/1 -> Switch2/1
  Constant2/1 -> Switch2/3, Switch1/1
  Data Type Conversion2/1 -> Switch1/3
  sawtooth generator/1(saw) -> Relational Operator3/2, Relational Operator2/2
  Gain1/1 -> Relational Operator3/1
  In1/1 -> Relational Operator2/1, Switch2/2, Switch1/2, Gain1/1
  Switch2/1 -> Out1/1
  Switch1/1 -> Out2/1

== system allmodes/battery controller /SUIM1/Subsystem1 ==
  In1 : Inport
  Integrator : Integrator
  ain9 : Gain  Gain=5  ParameterDataType=fixdt(1, 16)  ParameterScaling=2^0  OutDataType=fixdt(1, 16)  OutScaling=2^0
  Out1 : Outport
  wires:
  In1/1 -> ain9/1
  Integrator/1 -> Out1/1
  ain9/1 -> Integrator/1

== system allmodes/battery controller /SUIM1/Subsystem2 ==
  In1 : Inport
  Integrator : Integrator
  ain9 : Gain  Gain=5  ParameterDataType=fixdt(1, 16)  ParameterScaling=2^0  OutDataType=fixdt(1, 16)  OutScaling=2^0
  Out1 : Outport
  wires:
  ain9/1 -> Integrator/1
  Integrator/1 -> Out1/1
  In1/1 -> ain9/1

== system allmodes/battery controller /SUIM1/Subsystem3 ==
  In1 : Inport
  Integrator : Integrator
  ain9 : Gain  Gain=5  ParameterDataType=fixdt(1, 16)  ParameterScaling=2^0  OutDataType=fixdt(1, 16)  OutScaling=2^0
  Out1 : Outport
  wires:
  In1/1 -> ain9/1
  Integrator/1 -> Out1/1
  ain9/1 -> Integrator/1

== system allmodes/battery controller /v1/Subsystem ==
  In1 : Inport
  Enable : EnablePort
  Constant2 : Constant  Value=0  OutDataType=fixdt(1, 16)  OutScaling=2^0
  Data Type Conversion2 : DataTypeConversion  OutDataType=fixdt(1, 16)  OutScaling=2^0
  Data Type Conversion3 : DataTypeConversion  OutDataType=fixdt(1, 16)  OutScaling=2^0
  Gain1 : Gain  Gain=-1  ParameterDataType=fixdt(1, 16)  ParameterScaling=2^0  OutDataType=fixdt(1, 16)  OutScaling=2^0
  Relational Operator2 : RelationalOperator  Operator=>  LogicOutDataTypeMode=boolean  LogicDataType=fixdt(0, 8)  OutDataTypeStr=boolean
  Relational Operator3 : RelationalOperator  Operator=>  LogicOutDataTypeMode=boolean  LogicDataType=fixdt(0, 8)  OutDataTypeStr=boolean
  Switch1 : Switch  OutDataType=fixdt(1, 16)  OutScaling=2^0
  Switch2 : Switch  Criteria=u2 > Threshold  OutDataType=fixdt(1, 16)  OutScaling=2^0
  sawtooth generator : Subsystem  mask{fsw=5e3, vc=1}
      mask prompts: fsw "switching frequency"; vc "magnitude"
  Out1 : Outport
  Out2 : Outport  Port=2
  wires:
  Gain1/1 -> Relational Operator3/1
  sawtooth generator/1(saw) -> Relational Operator2/2, Relational Operator3/2
  Data Type Conversion2/1 -> Switch1/3
  Constant2/1 -> Switch1/1, Switch2/3
  Data Type Conversion3/1 -> Switch2/1
  Relational Operator2/1 -> Data Type Conversion3/1
  Relational Operator3/1 -> Data Type Conversion2/1
  In1/1 -> Gain1/1, Switch1/2, Switch2/2, Relational Operator2/1
  Switch2/1 -> Out1/1
  Switch1/1 -> Out2/1

== system allmodes/battery controller /v1/Subsystem1 ==
  In1 : Inport
  Integrator : Integrator
  ain9 : Gain  Gain=5  ParameterDataType=fixdt(1, 16)  ParameterScaling=2^0  OutDataType=fixdt(1, 16)  OutScaling=2^0
  Out1 : Outport
  wires:
  ain9/1 -> Integrator/1
  Integrator/1 -> Out1/1
  In1/1 -> ain9/1

== system allmodes/battery controller /v1/Subsystem2 ==
  In1 : Inport
  Integrator : Integrator
  ain9 : Gain  Gain=5  ParameterDataType=fixdt(1, 16)  ParameterScaling=2^0  OutDataType=fixdt(1, 16)  OutScaling=2^0
  Out1 : Outport
  wires:
  In1/1 -> ain9/1
  Integrator/1 -> Out1/1
  ain9/1 -> Integrator/1

== system allmodes/battery controller /v1/Subsystem3 ==
  In1 : Inport
  Integrator : Integrator
  ain9 : Gain  Gain=5  ParameterDataType=fixdt(1, 16)  ParameterScaling=2^0  OutDataType=fixdt(1, 16)  OutScaling=2^0
  Out1 : Outport
  wires:
  ain9/1 -> Integrator/1
  Integrator/1 -> Out1/1
  In1/1 -> ain9/1

== system allmodes/battery controller /v10/Subsystem ==
  In1 : Inport
  Enable : EnablePort
  Constant2 : Constant  Value=0  OutDataType=fixdt(1, 16)  OutScaling=2^0
  Data Type Conversion2 : DataTypeConversion  OutDataType=fixdt(1, 16)  OutScaling=2^0
  Data Type Conversion3 : DataTypeConversion  OutDataType=fixdt(1, 16)  OutScaling=2^0
  Gain1 : Gain  Gain=-1  ParameterDataType=fixdt(1, 16)  ParameterScaling=2^0  OutDataType=fixdt(1, 16)  OutScaling=2^0
  Relational Operator2 : RelationalOperator  Operator=>  LogicOutDataTypeMode=boolean  LogicDataType=fixdt(0, 8)  OutDataTypeStr=boolean
  Relational Operator3 : RelationalOperator  Operator=>  LogicOutDataTypeMode=boolean  LogicDataType=fixdt(0, 8)  OutDataTypeStr=boolean
  Switch1 : Switch  OutDataType=fixdt(1, 16)  OutScaling=2^0
  Switch2 : Switch  Criteria=u2 > Threshold  OutDataType=fixdt(1, 16)  OutScaling=2^0
  sawtooth generator : Subsystem  mask{fsw=5e3, vc=1}
      mask prompts: fsw "switching frequency"; vc "magnitude"
  Out1 : Outport
  Out2 : Outport  Port=2
  wires:
  Switch1/1 -> Out2/1
  Switch2/1 -> Out1/1
  In1/1 -> Relational Operator2/1, Switch2/2, Switch1/2, Gain1/1
  Relational Operator3/1 -> Data Type Conversion2/1
  Relational Operator2/1 -> Data Type Conversion3/1
  Data Type Conversion3/1 -> Switch2/1
  Constant2/1 -> Switch2/3, Switch1/1
  Data Type Conversion2/1 -> Switch1/3
  sawtooth generator/1(saw) -> Relational Operator3/2, Relational Operator2/2
  Gain1/1 -> Relational Operator3/1

== system allmodes/battery controller /v10/Subsystem1 ==
  In1 : Inport
  Integrator : Integrator
  ain9 : Gain  Gain=5  ParameterDataType=fixdt(1, 16)  ParameterScaling=2^0  OutDataType=fixdt(1, 16)  OutScaling=2^0
  Out1 : Outport
  wires:
  In1/1 -> ain9/1
  Integrator/1 -> Out1/1
  ain9/1 -> Integrator/1

== system allmodes/battery controller /v10/Subsystem2 ==
  In1 : Inport
  Integrator : Integrator
  ain9 : Gain  Gain=5  ParameterDataType=fixdt(1, 16)  ParameterScaling=2^0  OutDataType=fixdt(1, 16)  OutScaling=2^0
  Out1 : Outport
  wires:
  ain9/1 -> Integrator/1
  Integrator/1 -> Out1/1
  In1/1 -> ain9/1

== system allmodes/battery controller /v10/Subsystem3 ==
  In1 : Inport
  Integrator : Integrator
  ain9 : Gain  Gain=5  ParameterDataType=fixdt(1, 16)  ParameterScaling=2^0  OutDataType=fixdt(1, 16)  OutScaling=2^0
  Out1 : Outport
  wires:
  In1/1 -> ain9/1
  Integrator/1 -> Out1/1
  ain9/1 -> Integrator/1

== system allmodes/battery controller /v11/Subsystem ==
  In1 : Inport
  Enable : EnablePort
  Constant2 : Constant  Value=0  OutDataType=fixdt(1, 16)  OutScaling=2^0
  Data Type Conversion2 : DataTypeConversion  OutDataType=fixdt(1, 16)  OutScaling=2^0
  Data Type Conversion3 : DataTypeConversion  OutDataType=fixdt(1, 16)  OutScaling=2^0
  Gain1 : Gain  Gain=-1  ParameterDataType=fixdt(1, 16)  ParameterScaling=2^0  OutDataType=fixdt(1, 16)  OutScaling=2^0
  Relational Operator2 : RelationalOperator  Operator=>  LogicOutDataTypeMode=boolean  LogicDataType=fixdt(0, 8)  OutDataTypeStr=boolean
  Relational Operator3 : RelationalOperator  Operator=>  LogicOutDataTypeMode=boolean  LogicDataType=fixdt(0, 8)  OutDataTypeStr=boolean
  Switch1 : Switch  OutDataType=fixdt(1, 16)  OutScaling=2^0
  Switch2 : Switch  Criteria=u2 > Threshold  OutDataType=fixdt(1, 16)  OutScaling=2^0
  sawtooth generator : Subsystem  mask{fsw=5e3, vc=1}
      mask prompts: fsw "switching frequency"; vc "magnitude"
  Out1 : Outport
  Out2 : Outport  Port=2
  wires:
  Switch1/1 -> Out2/1
  Switch2/1 -> Out1/1
  In1/1 -> Relational Operator2/1, Switch2/2, Switch1/2, Gain1/1
  Relational Operator3/1 -> Data Type Conversion2/1
  Relational Operator2/1 -> Data Type Conversion3/1
  Data Type Conversion3/1 -> Switch2/1
  Constant2/1 -> Switch2/3, Switch1/1
  Data Type Conversion2/1 -> Switch1/3
  sawtooth generator/1(saw) -> Relational Operator3/2, Relational Operator2/2
  Gain1/1 -> Relational Operator3/1

== system allmodes/battery controller /v11/Subsystem1 ==
  In1 : Inport
  Integrator : Integrator
  ain9 : Gain  Gain=5  ParameterDataType=fixdt(1, 16)  ParameterScaling=2^0  OutDataType=fixdt(1, 16)  OutScaling=2^0
  Out1 : Outport
  wires:
  In1/1 -> ain9/1
  Integrator/1 -> Out1/1
  ain9/1 -> Integrator/1

== system allmodes/battery controller /v11/Subsystem2 ==
  In1 : Inport
  Integrator : Integrator
  ain9 : Gain  Gain=5  ParameterDataType=fixdt(1, 16)  ParameterScaling=2^0  OutDataType=fixdt(1, 16)  OutScaling=2^0
  Out1 : Outport
  wires:
  ain9/1 -> Integrator/1
  Integrator/1 -> Out1/1
  In1/1 -> ain9/1

== system allmodes/battery controller /v11/Subsystem3 ==
  In1 : Inport
  Integrator : Integrator
  ain9 : Gain  Gain=5  ParameterDataType=fixdt(1, 16)  ParameterScaling=2^0  OutDataType=fixdt(1, 16)  OutScaling=2^0
  Out1 : Outport
  wires:
  In1/1 -> ain9/1
  Integrator/1 -> Out1/1
  ain9/1 -> Integrator/1

== system allmodes/battery controller /v12/Subsystem ==
  In1 : Inport
  Enable : EnablePort
  Constant2 : Constant  Value=0  OutDataType=fixdt(1, 16)  OutScaling=2^0
  Data Type Conversion2 : DataTypeConversion  OutDataType=fixdt(1, 16)  OutScaling=2^0
  Data Type Conversion3 : DataTypeConversion  OutDataType=fixdt(1, 16)  OutScaling=2^0
  Gain1 : Gain  Gain=-1  ParameterDataType=fixdt(1, 16)  ParameterScaling=2^0  OutDataType=fixdt(1, 16)  OutScaling=2^0
  Relational Operator2 : RelationalOperator  Operator=>  LogicOutDataTypeMode=boolean  LogicDataType=fixdt(0, 8)  OutDataTypeStr=boolean
  Relational Operator3 : RelationalOperator  Operator=>  LogicOutDataTypeMode=boolean  LogicDataType=fixdt(0, 8)  OutDataTypeStr=boolean
  Switch1 : Switch  OutDataType=fixdt(1, 16)  OutScaling=2^0
  Switch2 : Switch  Criteria=u2 > Threshold  OutDataType=fixdt(1, 16)  OutScaling=2^0
  sawtooth generator : Subsystem  mask{fsw=5e3, vc=1}
      mask prompts: fsw "switching frequency"; vc "magnitude"
  Out1 : Outport
  Out2 : Outport  Port=2
  wires:
  Switch1/1 -> Out2/1
  Switch2/1 -> Out1/1
  In1/1 -> Relational Operator2/1, Switch2/2, Switch1/2, Gain1/1
  Relational Operator3/1 -> Data Type Conversion2/1
  Relational Operator2/1 -> Data Type Conversion3/1
  Data Type Conversion3/1 -> Switch2/1
  Constant2/1 -> Switch2/3, Switch1/1
  Data Type Conversion2/1 -> Switch1/3
  sawtooth generator/1(saw) -> Relational Operator3/2, Relational Operator2/2
  Gain1/1 -> Relational Operator3/1

== system allmodes/battery controller /v12/Subsystem1 ==
  In1 : Inport
  Integrator : Integrator
  ain9 : Gain  Gain=5  ParameterDataType=fixdt(1, 16)  ParameterScaling=2^0  OutDataType=fixdt(1, 16)  OutScaling=2^0
  Out1 : Outport
  wires:
  In1/1 -> ain9/1
  Integrator/1 -> Out1/1
  ain9/1 -> Integrator/1

== system allmodes/battery controller /v12/Subsystem2 ==
  In1 : Inport
  Integrator : Integrator
  ain9 : Gain  Gain=5  ParameterDataType=fixdt(1, 16)  ParameterScaling=2^0  OutDataType=fixdt(1, 16)  OutScaling=2^0
  Out1 : Outport
  wires:
  ain9/1 -> Integrator/1
  Integrator/1 -> Out1/1
  In1/1 -> ain9/1

== system allmodes/battery controller /v12/Subsystem3 ==
  In1 : Inport
  Integrator : Integrator
  ain9 : Gain  Gain=5  ParameterDataType=fixdt(1, 16)  ParameterScaling=2^0  OutDataType=fixdt(1, 16)  OutScaling=2^0
  Out1 : Outport
  wires:
  In1/1 -> ain9/1
  Integrator/1 -> Out1/1
  ain9/1 -> Integrator/1

== system allmodes/battery controller /v13/Subsystem ==
  In1 : Inport
  Enable : EnablePort
  Constant2 : Constant  Value=0  OutDataType=fixdt(1, 16)  OutScaling=2^0
  Data Type Conversion2 : DataTypeConversion  OutDataType=fixdt(1, 16)  OutScaling=2^0
  Data Type Conversion3 : DataTypeConversion  OutDataType=fixdt(1, 16)  OutScaling=2^0
  Gain1 : Gain  Gain=-1  ParameterDataType=fixdt(1, 16)  ParameterScaling=2^0  OutDataType=fixdt(1, 16)  OutScaling=2^0
  Relational Operator2 : RelationalOperator  Operator=>  LogicOutDataTypeMode=boolean  LogicDataType=fixdt(0, 8)  OutDataTypeStr=boolean
  Relational Operator3 : RelationalOperator  Operator=>  LogicOutDataTypeMode=boolean  LogicDataType=fixdt(0, 8)  OutDataTypeStr=boolean
  Switch1 : Switch  OutDataType=fixdt(1, 16)  OutScaling=2^0
  Switch2 : Switch  Criteria=u2 > Threshold  OutDataType=fixdt(1, 16)  OutScaling=2^0
  sawtooth generator : Subsystem  mask{fsw=5e3, vc=1}
      mask prompts: fsw "switching frequency"; vc "magnitude"
  Out1 : Outport
  Out2 : Outport  Port=2
  wires:
  Switch1/1 -> Out2/1
  Switch2/1 -> Out1/1
  In1/1 -> Relational Operator2/1, Switch2/2, Switch1/2, Gain1/1
  Relational Operator3/1 -> Data Type Conversion2/1
  Relational Operator2/1 -> Data Type Conversion3/1
  Data Type Conversion3/1 -> Switch2/1
  Constant2/1 -> Switch2/3, Switch1/1
  Data Type Conversion2/1 -> Switch1/3
  sawtooth generator/1(saw) -> Relational Operator3/2, Relational Operator2/2
  Gain1/1 -> Relational Operator3/1

== system allmodes/battery controller /v13/Subsystem1 ==
  In1 : Inport
  Integrator : Integrator
  ain9 : Gain  Gain=5  ParameterDataType=fixdt(1, 16)  ParameterScaling=2^0  OutDataType=fixdt(1, 16)  OutScaling=2^0
  Out1 : Outport
  wires:
  In1/1 -> ain9/1
  Integrator/1 -> Out1/1
  ain9/1 -> Integrator/1

== system allmodes/battery controller /v13/Subsystem2 ==
  In1 : Inport
  Integrator : Integrator
  ain9 : Gain  Gain=5  ParameterDataType=fixdt(1, 16)  ParameterScaling=2^0  OutDataType=fixdt(1, 16)  OutScaling=2^0
  Out1 : Outport
  wires:
  ain9/1 -> Integrator/1
  Integrator/1 -> Out1/1
  In1/1 -> ain9/1

== system allmodes/battery controller /v13/Subsystem3 ==
  In1 : Inport
  Integrator : Integrator
  ain9 : Gain  Gain=5  ParameterDataType=fixdt(1, 16)  ParameterScaling=2^0  OutDataType=fixdt(1, 16)  OutScaling=2^0
  Out1 : Outport
  wires:
  In1/1 -> ain9/1
  Integrator/1 -> Out1/1
  ain9/1 -> Integrator/1

== system allmodes/battery controller /v14/Subsystem ==
  In1 : Inport
  Enable : EnablePort
  Constant2 : Constant  Value=0  OutDataType=fixdt(1, 16)  OutScaling=2^0
  Data Type Conversion2 : DataTypeConversion  OutDataType=fixdt(1, 16)  OutScaling=2^0
  Data Type Conversion3 : DataTypeConversion  OutDataType=fixdt(1, 16)  OutScaling=2^0
  Gain1 : Gain  Gain=-1  ParameterDataType=fixdt(1, 16)  ParameterScaling=2^0  OutDataType=fixdt(1, 16)  OutScaling=2^0
  Relational Operator2 : RelationalOperator  Operator=>  LogicOutDataTypeMode=boolean  LogicDataType=fixdt(0, 8)  OutDataTypeStr=boolean
  Relational Operator3 : RelationalOperator  Operator=>  LogicOutDataTypeMode=boolean  LogicDataType=fixdt(0, 8)  OutDataTypeStr=boolean
  Switch1 : Switch  OutDataType=fixdt(1, 16)  OutScaling=2^0
  Switch2 : Switch  Criteria=u2 > Threshold  OutDataType=fixdt(1, 16)  OutScaling=2^0
  sawtooth generator : Subsystem  mask{fsw=5e3, vc=1}
      mask prompts: fsw "switching frequency"; vc "magnitude"
  Out1 : Outport
  Out2 : Outport  Port=2
  wires:
  Switch1/1 -> Out2/1
  Switch2/1 -> Out1/1
  In1/1 -> Relational Operator2/1, Switch2/2, Switch1/2, Gain1/1
  Relational Operator3/1 -> Data Type Conversion2/1
  Relational Operator2/1 -> Data Type Conversion3/1
  Data Type Conversion3/1 -> Switch2/1
  Constant2/1 -> Switch2/3, Switch1/1
  Data Type Conversion2/1 -> Switch1/3
  sawtooth generator/1(saw) -> Relational Operator3/2, Relational Operator2/2
  Gain1/1 -> Relational Operator3/1

== system allmodes/battery controller /v14/Subsystem1 ==
  In1 : Inport
  Integrator : Integrator
  ain9 : Gain  Gain=5  ParameterDataType=fixdt(1, 16)  ParameterScaling=2^0  OutDataType=fixdt(1, 16)  OutScaling=2^0
  Out1 : Outport
  wires:
  In1/1 -> ain9/1
  Integrator/1 -> Out1/1
  ain9/1 -> Integrator/1

== system allmodes/battery controller /v14/Subsystem2 ==
  In1 : Inport
  Integrator : Integrator
  ain9 : Gain  Gain=5  ParameterDataType=fixdt(1, 16)  ParameterScaling=2^0  OutDataType=fixdt(1, 16)  OutScaling=2^0
  Out1 : Outport
  wires:
  ain9/1 -> Integrator/1
  Integrator/1 -> Out1/1
  In1/1 -> ain9/1

== system allmodes/battery controller /v14/Subsystem3 ==
  In1 : Inport
  Integrator : Integrator
  ain9 : Gain  Gain=5  ParameterDataType=fixdt(1, 16)  ParameterScaling=2^0  OutDataType=fixdt(1, 16)  OutScaling=2^0
  Out1 : Outport
  wires:
  In1/1 -> ain9/1
  Integrator/1 -> Out1/1
  ain9/1 -> Integrator/1

== system allmodes/battery controller /v15/Subsystem ==
  In1 : Inport
  Enable : EnablePort
  Constant2 : Constant  Value=0  OutDataType=fixdt(1, 16)  OutScaling=2^0
  Data Type Conversion2 : DataTypeConversion  OutDataType=fixdt(1, 16)  OutScaling=2^0
  Data Type Conversion3 : DataTypeConversion  OutDataType=fixdt(1, 16)  OutScaling=2^0
  Gain1 : Gain  Gain=-1  ParameterDataType=fixdt(1, 16)  ParameterScaling=2^0  OutDataType=fixdt(1, 16)  OutScaling=2^0
  Relational Operator2 : RelationalOperator  Operator=>  LogicOutDataTypeMode=boolean  LogicDataType=fixdt(0, 8)  OutDataTypeStr=boolean
  Relational Operator3 : RelationalOperator  Operator=>  LogicOutDataTypeMode=boolean  LogicDataType=fixdt(0, 8)  OutDataTypeStr=boolean
  Switch1 : Switch  OutDataType=fixdt(1, 16)  OutScaling=2^0
  Switch2 : Switch  Criteria=u2 > Threshold  OutDataType=fixdt(1, 16)  OutScaling=2^0
  sawtooth generator : Subsystem  mask{fsw=5e3, vc=1}
      mask prompts: fsw "switching frequency"; vc "magnitude"
  Out1 : Outport
  Out2 : Outport  Port=2
  wires:
  Switch1/1 -> Out2/1
  Switch2/1 -> Out1/1
  In1/1 -> Relational Operator2/1, Switch2/2, Switch1/2, Gain1/1
  Relational Operator3/1 -> Data Type Conversion2/1
  Relational Operator2/1 -> Data Type Conversion3/1
  Data Type Conversion3/1 -> Switch2/1
  Constant2/1 -> Switch2/3, Switch1/1
  Data Type Conversion2/1 -> Switch1/3
  sawtooth generator/1(saw) -> Relational Operator3/2, Relational Operator2/2
  Gain1/1 -> Relational Operator3/1

== system allmodes/battery controller /v15/Subsystem1 ==
  In1 : Inport
  Integrator : Integrator
  ain9 : Gain  Gain=5  ParameterDataType=fixdt(1, 16)  ParameterScaling=2^0  OutDataType=fixdt(1, 16)  OutScaling=2^0
  Out1 : Outport
  wires:
  In1/1 -> ain9/1
  Integrator/1 -> Out1/1
  ain9/1 -> Integrator/1

== system allmodes/battery controller /v15/Subsystem2 ==
  In1 : Inport
  Integrator : Integrator
  ain9 : Gain  Gain=5  ParameterDataType=fixdt(1, 16)  ParameterScaling=2^0  OutDataType=fixdt(1, 16)  OutScaling=2^0
  Out1 : Outport
  wires:
  ain9/1 -> Integrator/1
  Integrator/1 -> Out1/1
  In1/1 -> ain9/1

== system allmodes/battery controller /v15/Subsystem3 ==
  In1 : Inport
  Integrator : Integrator
  ain9 : Gain  Gain=5  ParameterDataType=fixdt(1, 16)  ParameterScaling=2^0  OutDataType=fixdt(1, 16)  OutScaling=2^0
  Out1 : Outport
  wires:
  In1/1 -> ain9/1
  Integrator/1 -> Out1/1
  ain9/1 -> Integrator/1
